simulink model "SS_1115"  (R2014a)
settings: Solver=FixedStepDiscrete  StartTime=0.0  StopTime=5  FixedStep=0.0005  RelTol=1e-3
values from neighbouring files (symbols this model uses):
  APS_High_null = ecucoder_cal(APS_High_null)    [SS.m]
  APS_High_x = ecucoder_cal(APS_High_x)    [SS.m]
  APS_High_y = ecucoder_cal(APS_High_y)    [SS.m]
  APS_Low_null = ecucoder_cal(APS_Low_null)    [SS.m]
  APS_low_x = ecucoder_cal(APS_low_x)    [SS.m]
  APS_low_y = ecucoder_cal(APS_low_y)    [SS.m]
  BrakeSignal_cal = ecucoder_cal(BrakeSignal_cal)    [SS.m]
  CustomReduceFactor_cal = ecucoder_cal(CustomReduceFactor_cal)    [SS.m]
  Differential_cal = ecucoder_cal(Differential_cal)    [SS.m]
  LowSOCWarning_cal = ecucoder_cal(LowSOCWarning_cal)    [SS.m]
  MotorTemperatureHigh_cal = ecucoder_cal(MotorTemperatureHigh_cal)    [SS.m]
  MotorTemperatureLow_cal = ecucoder_cal(MotorTemperatureLow_cal)    [SS.m]
  OilPressure_x = ecucoder_cal(OilPressure_x)    [SS.m]
  OilPressure_y = ecucoder_cal(OilPressure_y)    [SS.m]
  PowerBias_cal = ecucoder_cal(PowerBias_cal)    [SS.m]
  SpeedLimitFactor_x = ecucoder_cal(SpeedLimitFactor_x)    [SS.m]
  SpeedLimitFactor_y = ecucoder_cal(SpeedLimitFactor_y)    [SS.m]
  SteerAngle_x = ecucoder_cal(SteerAngle_x)    [SS.m]
  SteerAngle_y = ecucoder_cal(SteerAngle_y)    [SS.m]
  SteerThresholdHigh_cal = ecucoder_cal(SteerThresholdHigh_cal)    [SS.m]
  SteerThresholdLow_cal = ecucoder_cal(SteerThresholdLow_cal)    [SS.m]
  TorqueLimitNegativ_cal = ecucoder_cal(TorqueLimitNegativ_cal)    [SS.m]
  TorqueLimitPositiv_cal = ecucoder_cal(TorqueLimitPositiv_cal)    [SS.m]
libraries: simulink x101, ec55xxlib x32
(part 3 of 3)

== system SS_1115/VCU_MCU/Enabled Subsystem/Torquearrengement/AMK1 ==
  v : Inport
  Taim : Inport  Port=2
  1-D Lookup Table : Lookup_n-D  NumberOfTableDimensions=1  BreakpointsForDimension1=[0 13000 14000 15000 16000 17000 18000 19000]  Table=[21 21 20 17 16 13 8 0]  ExtrapMethod=Clip  InternalRulePriority=Speed  RndMeth=Simplest  InputSameDT=on
  Constant : Constant  Value=0.0098  SampleTime=-1
  Divide : Product  Inputs=*/  OutDataTypeStr=single
  Divide1 : Product  Inputs=*/  OutDataTypeStr=single
  Saturation : Saturate  UpperLimit=2000  LowerLimit=0
  "ReduceFactor " : Outport
  wires:
  v/1 -> 1-D Lookup Table/1
  1-D Lookup Table/1 -> Divide/1
  Constant/1 -> Divide/2
  Divide/1 -> Saturation/1
  Taim/1 -> Divide1/2
  Divide1/1 -> "ReduceFactor "/1
  Saturation/1 -> Divide1/1

== system SS_1115/VCU_MCU/Enabled Subsystem/Torquearrengement/AMK2 ==
  v : Inport
  Taim : Inport  Port=2
  1-D Lookup Table : Lookup_n-D  NumberOfTableDimensions=1  BreakpointsForDimension1=[0 13000 14000 15000 16000 17000 18000 19000]  Table=[21 21 20 17 16 13 8 0]  ExtrapMethod=Clip  InternalRulePriority=Speed  RndMeth=Simplest  InputSameDT=on
  Constant : Constant  Value=0.0098  SampleTime=-1
  Divide : Product  Inputs=*/  OutDataTypeStr=single
  Divide1 : Product  Inputs=*/  OutDataTypeStr=single
  Saturation : Saturate  UpperLimit=2000  LowerLimit=0
  "ReduceFactor " : Outport
  wires:
  v/1 -> 1-D Lookup Table/1
  1-D Lookup Table/1 -> Divide/1
  Constant/1 -> Divide/2
  Divide/1 -> Saturation/1
  Taim/1 -> Divide1/2
  Divide1/1 -> "ReduceFactor "/1
  Saturation/1 -> Divide1/1

== system SS_1115/VCU_MCU/Enabled Subsystem/Torquearrengement/AMK3 ==
  v : Inport
  Taim : Inport  Port=2
  1-D Lookup Table : Lookup_n-D  NumberOfTableDimensions=1  BreakpointsForDimension1=[0 13000 14000 15000 16000 17000 18000 19000]  Table=[21 21 20 17 16 13 8 0]  ExtrapMethod=Clip  InternalRulePriority=Speed  RndMeth=Simplest  InputSameDT=on
  Constant : Constant  Value=0.0098  SampleTime=-1
  Divide : Product  Inputs=*/  OutDataTypeStr=single
  Divide1 : Product  Inputs=*/  OutDataTypeStr=single
  Saturation : Saturate  UpperLimit=2000  LowerLimit=0
  "ReduceFactor " : Outport
  wires:
  v/1 -> 1-D Lookup Table/1
  1-D Lookup Table/1 -> Divide/1
  Constant/1 -> Divide/2
  Divide/1 -> Saturation/1
  Taim/1 -> Divide1/2
  Divide1/1 -> "ReduceFactor "/1
  Saturation/1 -> Divide1/1

== system SS_1115/VCU_MCU/Enabled Subsystem/Torquearrengement/AMK4 ==
  v : Inport
  Taim : Inport  Port=2
  1-D Lookup Table : Lookup_n-D  NumberOfTableDimensions=1  BreakpointsForDimension1=[0 13000 14000 15000 16000 17000 18000 19000]  Table=[21 21 20 17 16 13 8 0]  ExtrapMethod=Clip  InternalRulePriority=Speed  RndMeth=Simplest  InputSameDT=on
  Constant : Constant  Value=0.0098  SampleTime=-1
  Divide : Product  Inputs=*/  OutDataTypeStr=single
  Divide1 : Product  Inputs=*/  OutDataTypeStr=single
  Saturation : Saturate  UpperLimit=2000  LowerLimit=0
  "ReduceFactor " : Outport
  wires:
  v/1 -> 1-D Lookup Table/1
  1-D Lookup Table/1 -> Divide/1
  Constant/1 -> Divide/2
  Divide/1 -> Saturation/1
  Taim/1 -> Divide1/2
  Divide1/1 -> "ReduceFactor "/1
  Saturation/1 -> Divide1/1

== system SS_1115/VCU_MCU/Enabled Subsystem/Torquearrengement/Differential_ ==
  note: 暂定转角负为左转，正为右转
  note: T1左前 T2右前 T3左后 T4右后
  TIT2 : Inport
  T3T4 : Inport  Port=2
  CAN0333OK : Inport  Port=3
  DifferentialUplimit : Inport  Port=4
  SteerAngleInDegree : Inport  Port=5
  Chart1 : Stateflow chart  TreatAsAtomicUnit=on
  Chart2 : Stateflow chart  TreatAsAtomicUnit=on
  Compare To Constant : simulink/Logic and Bit Operations/Compare To Constant  relop===  const=1  OutDataTypeStr=boolean
  Constant : Constant  Value=SteerThresholdLow_cal  SampleTime=-1
  Constant1 : Constant  Value=SteerThresholdHigh_cal  SampleTime=-1
  Data Type Conversion : DataTypeConversion  OutDataTypeStr=int16
  Data Type Conversion1 : DataTypeConversion  OutDataTypeStr=int16
  Switch : Switch  Criteria=u2 > Threshold
  Unit Delay : UnitDelay  InitialCondition=Differential_cal  SampleTime=-1
  Watchup-Table : Subsystem  TreatAsAtomicUnit=on
  T1 : Outport
  T2 : Outport  Port=2
  T3 : Outport  Port=3
  T4 : Outport  Port=4
  Differential UpLimit : Outport  Port=5
  wires:
  TIT2/1 -> Chart2/1(Sumof2Wheels)
  T3T4/1 -> Chart1/1(Sumof2Wheels)
  CAN0333OK/1 -> Compare To Constant/1
  DifferentialUplimit/1 -> Switch/1
  Unit Delay/1 -> Switch/3
  Compare To Constant/1 -> Switch/2
  Switch/1 -> Unit Delay/1, Watchup-Table/1(DifferentialUpLimit), Differential UpLimit/1  "DifferentialLimit_mea"
  Watchup-Table/1(Differential) -> [DiffFactorRT]  "DiffFactorRT_mea"
  SteerAngleInDegree/1 -> Chart2/2(SteerAngle), Chart1/2(SteerAngle), Watchup-Table/2(SteerAngle)
  Constant/1 -> Data Type Conversion/1
  Data Type Conversion/1 -> Watchup-Table/3(AngleTreshholdLow)  "AngleThresholdLow_mea"
  Constant1/1 -> Data Type Conversion1/1
  Data Type Conversion1/1 -> Watchup-Table/4(AngleTreshholdHigh)  "AngleThresholdHigh_mea"
  [DiffFactorRT] -> Chart2/3(DiffFactorRT)
  Chart2/1(Power2Left) -> T1/1
  Chart2/2(Power2Right) -> T2/1
  Chart1/1(Power2Left) -> T3/1
  Chart1/2(Power2Right) -> T4/1
  [DiffFactorRT] -> Chart1/3(DiffFactorRT)

== system SS_1115/VCU_MCU/Enabled Subsystem/Torquearrengement/Power Cal1 ==
  aim_torque : Inport
  "rotate speed " : Inport  Port=2
  Gain : Gain  Gain=0.0098
  Gain1 : Gain  Gain=1/9549  ParamDataTypeStr=single
  Product : Product  OutDataTypeStr=single
  power : Outport
  wires:
  aim_torque/1 -> Gain/1
  Gain/1 -> Product/1
  "rotate speed "/1 -> Product/2
  Product/1 -> Gain1/1
  Gain1/1 -> power/1

== system SS_1115/VCU_MCU/Enabled Subsystem/Torquearrengement/Power Cal2 ==
  aim_torque : Inport
  "rotate speed " : Inport  Port=2
  Gain : Gain  Gain=0.0098
  Gain1 : Gain  Gain=1/9549  ParamDataTypeStr=single
  Product : Product  OutDataTypeStr=single
  power : Outport
  wires:
  aim_torque/1 -> Gain/1
  Gain/1 -> Product/1
  "rotate speed "/1 -> Product/2
  Product/1 -> Gain1/1
  Gain1/1 -> power/1

== system SS_1115/VCU_MCU/Enabled Subsystem/Torquearrengement/Power Cal3 ==
  aim_torque : Inport
  "rotate speed " : Inport  Port=2
  Gain : Gain  Gain=0.0098
  Gain1 : Gain  Gain=1/9549  ParamDataTypeStr=single
  Product : Product  OutDataTypeStr=single
  power : Outport
  wires:
  aim_torque/1 -> Gain/1
  Gain/1 -> Product/1
  "rotate speed "/1 -> Product/2
  Product/1 -> Gain1/1
  Gain1/1 -> power/1

== system SS_1115/VCU_MCU/Enabled Subsystem/Torquearrengement/Power Cal4 ==
  aim_torque : Inport
  "rotate speed " : Inport  Port=2
  Gain : Gain  Gain=0.0098
  Gain1 : Gain  Gain=1/9549  ParamDataTypeStr=single
  Product : Product  OutDataTypeStr=single
  power : Outport
  wires:
  aim_torque/1 -> Gain/1
  Gain/1 -> Product/1
  "rotate speed "/1 -> Product/2
  Product/1 -> Gain1/1
  Gain1/1 -> power/1

== system SS_1115/VCU_MCU/Enabled Subsystem/Torquearrengement/PowerBias_ ==
  TqSum : Inport
  PowerBias : Inport  Port=2
  CAN0333OK : Inport  Port=3
  Add : Sum  Inputs=+-
  Compare To Constant : simulink/Logic and Bit Operations/Compare To Constant  relop===  const=1  OutDataTypeStr=boolean
  Constant2 : Constant  OutDataTypeStr=single  SampleTime=-1
  Gain : Gain  Gain=80
  Product : Product
  Product1 : Product
  Saturation : Saturate  UpperLimit=1  LowerLimit=0  LinearizeAsGain=off
  Saturation1 : Saturate  UpperLimit=1  LowerLimit=0  LinearizeAsGain=off
  Switch : Switch  Criteria=u2 > Threshold
  Unit Delay : UnitDelay  InitialCondition=PowerBias_cal  SampleTime=-1
  T1T2 : Outport
  T3T4 : Outport  Port=2
  "PowerBias " : Outport  Port=3
  wires:
  TqSum/1 -> Gain/1
  Product/1 -> T1T2/1
  Product1/1 -> T3T4/1
  Add/1 -> Saturation1/1
  [PowerBias] -> Add/2
  Constant2/1 -> Add/1
  CAN0333OK/1 -> Compare To Constant/1
  PowerBias/1 -> Switch/1
  Switch/1 -> [PowerBias], Unit Delay/1
  Unit Delay/1 -> Switch/3
  Compare To Constant/1 -> Switch/2
  [PowerBias] -> "PowerBias "/1
  Gain/1 -> Product1/2, Product/2
  [PowerBias] -> Saturation/1
  Saturation/1 -> Product/1  "FrontPowerBias_mea"
  Saturation1/1 -> Product1/1  "RearPowerBias_mea"

== system SS_1115/HardWare_Input/In1_Message/Function-Call Subsystem/Subsystem1/Subsystem ==
  In1 : Inport
  Bitwise Operator : simulink/Logic and Bit Operations/Bitwise Operator  logicop=AND  UseBitMask=on  BitMask=bin2dec('00000001')  BitMaskRealWorld=Stored Integer
  Bitwise Operator1 : simulink/Logic and Bit Operations/Bitwise Operator  logicop=AND  UseBitMask=on  BitMask=bin2dec('00000010')  BitMaskRealWorld=Stored Integer
  Bitwise Operator2 : simulink/Logic and Bit Operations/Bitwise Operator  logicop=AND  UseBitMask=on  BitMask=bin2dec('00001000')  BitMaskRealWorld=Stored Integer
  Bitwise Operator3 : simulink/Logic and Bit Operations/Bitwise Operator  logicop=AND  UseBitMask=on  BitMask=bin2dec('00100000')  BitMaskRealWorld=Stored Integer
  Shift Arithmetic1 : ArithShift  BitShiftNumber=3  BitShiftDirection=Right
  Shift Arithmetic2 : ArithShift  BitShiftNumber=1  BitShiftDirection=Right
  Shift Arithmetic3 : ArithShift  BitShiftNumber=5  BitShiftDirection=Right
  AMK_bSystemReady : Outport
  AMK_bError : Outport  Port=2
  AMK_bQuitDcOn : Outport  Port=3
  AMK_bQuitInverterOn : Outport  Port=4
  wires:
  Bitwise Operator1/1 -> Shift Arithmetic2/1
  Bitwise Operator/1 -> AMK_bSystemReady/1
  In1/1 -> Bitwise Operator3/1, Bitwise Operator2/1, Bitwise Operator1/1, Bitwise Operator/1
  Shift Arithmetic2/1 -> AMK_bError/1
  Bitwise Operator2/1 -> Shift Arithmetic1/1
  Shift Arithmetic1/1 -> AMK_bQuitDcOn/1
  Bitwise Operator3/1 -> Shift Arithmetic3/1
  Shift Arithmetic3/1 -> AMK_bQuitInverterOn/1

== system SS_1115/HardWare_Input/In2_Message/Function-Call Subsystem/Subsystem1/Subsystem ==
  In1 : Inport
  Bitwise Operator : simulink/Logic and Bit Operations/Bitwise Operator  logicop=AND  UseBitMask=on  BitMask=bin2dec('00000001')  BitMaskRealWorld=Stored Integer
  Bitwise Operator1 : simulink/Logic and Bit Operations/Bitwise Operator  logicop=AND  UseBitMask=on  BitMask=bin2dec('00000010')  BitMaskRealWorld=Stored Integer
  Bitwise Operator2 : simulink/Logic and Bit Operations/Bitwise Operator  logicop=AND  UseBitMask=on  BitMask=bin2dec('00001000')  BitMaskRealWorld=Stored Integer
  Bitwise Operator3 : simulink/Logic and Bit Operations/Bitwise Operator  logicop=AND  UseBitMask=on  BitMask=bin2dec('00100000')  BitMaskRealWorld=Stored Integer
  Shift Arithmetic1 : ArithShift  BitShiftNumber=3  BitShiftDirection=Right
  Shift Arithmetic2 : ArithShift  BitShiftNumber=1  BitShiftDirection=Right
  Shift Arithmetic3 : ArithShift  BitShiftNumber=5  BitShiftDirection=Right
  AMK_bSystemReady : Outport
  AMK_bError : Outport  Port=2
  AMK_bQuitDcOn : Outport  Port=3
  AMK_bQuitInverterOn : Outport  Port=4
  wires:
  Bitwise Operator1/1 -> Shift Arithmetic2/1
  Bitwise Operator/1 -> AMK_bSystemReady/1
  In1/1 -> Bitwise Operator3/1, Bitwise Operator2/1, Bitwise Operator1/1, Bitwise Operator/1
  Shift Arithmetic2/1 -> AMK_bError/1
  Bitwise Operator2/1 -> Shift Arithmetic1/1
  Shift Arithmetic1/1 -> AMK_bQuitDcOn/1
  Bitwise Operator3/1 -> Shift Arithmetic3/1
  Shift Arithmetic3/1 -> AMK_bQuitInverterOn/1

== system SS_1115/HardWare_Input/In3_Message/Function-Call Subsystem/Subsystem1/Subsystem ==
  In1 : Inport
  Bitwise Operator : simulink/Logic and Bit Operations/Bitwise Operator  logicop=AND  UseBitMask=on  BitMask=bin2dec('00000001')  BitMaskRealWorld=Stored Integer
  Bitwise Operator1 : simulink/Logic and Bit Operations/Bitwise Operator  logicop=AND  UseBitMask=on  BitMask=bin2dec('00000010')  BitMaskRealWorld=Stored Integer
  Bitwise Operator2 : simulink/Logic and Bit Operations/Bitwise Operator  logicop=AND  UseBitMask=on  BitMask=bin2dec('00001000')  BitMaskRealWorld=Stored Integer
  Bitwise Operator3 : simulink/Logic and Bit Operations/Bitwise Operator  logicop=AND  UseBitMask=on  BitMask=bin2dec('00100000')  BitMaskRealWorld=Stored Integer
  Shift Arithmetic1 : ArithShift  BitShiftNumber=3  BitShiftDirection=Right
  Shift Arithmetic2 : ArithShift  BitShiftNumber=1  BitShiftDirection=Right
  Shift Arithmetic3 : ArithShift  BitShiftNumber=5  BitShiftDirection=Right
  AMK_bSystemReady : Outport
  AMK_bError : Outport  Port=2
  AMK_bQuitDcOn : Outport  Port=3
  AMK_bQuitInverterOn : Outport  Port=4
  wires:
  Bitwise Operator1/1 -> Shift Arithmetic2/1
  Bitwise Operator/1 -> AMK_bSystemReady/1
  In1/1 -> Bitwise Operator3/1, Bitwise Operator2/1, Bitwise Operator1/1, Bitwise Operator/1
  Shift Arithmetic2/1 -> AMK_bError/1
  Bitwise Operator2/1 -> Shift Arithmetic1/1
  Shift Arithmetic1/1 -> AMK_bQuitDcOn/1
  Bitwise Operator3/1 -> Shift Arithmetic3/1
  Shift Arithmetic3/1 -> AMK_bQuitInverterOn/1

== system SS_1115/HardWare_Input/In4_Message/Function-Call Subsystem/Subsystem1/Subsystem ==
  In1 : Inport
  Bitwise Operator : simulink/Logic and Bit Operations/Bitwise Operator  logicop=AND  UseBitMask=on  BitMask=bin2dec('00000001')  BitMaskRealWorld=Stored Integer
  Bitwise Operator1 : simulink/Logic and Bit Operations/Bitwise Operator  logicop=AND  UseBitMask=on  BitMask=bin2dec('00000010')  BitMaskRealWorld=Stored Integer
  Bitwise Operator2 : simulink/Logic and Bit Operations/Bitwise Operator  logicop=AND  UseBitMask=on  BitMask=bin2dec('00001000')  BitMaskRealWorld=Stored Integer
  Bitwise Operator3 : simulink/Logic and Bit Operations/Bitwise Operator  logicop=AND  UseBitMask=on  BitMask=bin2dec('00100000')  BitMaskRealWorld=Stored Integer
  Shift Arithmetic1 : ArithShift  BitShiftNumber=3  BitShiftDirection=Right
  Shift Arithmetic2 : ArithShift  BitShiftNumber=1  BitShiftDirection=Right
  Shift Arithmetic3 : ArithShift  BitShiftNumber=5  BitShiftDirection=Right
  AMK_bSystemReady : Outport
  AMK_bError : Outport  Port=2
  AMK_bQuitDcOn : Outport  Port=3
  AMK_bQuitInverterOn : Outport  Port=4
  wires:
  Bitwise Operator1/1 -> Shift Arithmetic2/1
  Bitwise Operator/1 -> AMK_bSystemReady/1
  In1/1 -> Bitwise Operator3/1, Bitwise Operator2/1, Bitwise Operator1/1, Bitwise Operator/1
  Shift Arithmetic2/1 -> AMK_bError/1
  Bitwise Operator2/1 -> Shift Arithmetic1/1
  Shift Arithmetic1/1 -> AMK_bQuitDcOn/1
  Bitwise Operator3/1 -> Shift Arithmetic3/1
  Shift Arithmetic3/1 -> AMK_bQuitInverterOn/1

== system SS_1115/VCU_MCU/Enabled Subsystem/Torquearrengement/Differential_/Watchup-Table ==
  DifferentialUpLimit : Inport
  SteerAngle : Inport  Port=2
  AngleTreshholdLow : Inport  Port=3
  AngleTreshholdHigh : Inport  Port=4
  Abs : Abs
  Chart : Stateflow chart  TreatAsAtomicUnit=on
  Saturation : Saturate  UpperLimit=1  LowerLimit=0  LinearizeAsGain=off
  Differential : Outport
  wires:
  DifferentialUpLimit/1 -> Chart/1(DiffLimit)
  SteerAngle/1 -> Abs/1
  AngleTreshholdHigh/1 -> Chart/4(ThresholdHigh)
  AngleTreshholdLow/1 -> Chart/3(ThresholdLow)
  Chart/1(DiffFactor) -> Saturation/1
  Abs/1 -> Chart/2(SteerAngle)
  Saturation/1 -> Differential/1

== stateflow chart SS_1115/VCU_MCU/Enabled Subsystem/Chart1 ==
  state Normal
    entry:
    Logicvalue = single(1);
  state TimeCounting
    entry:
    Logicvalue = single(1);
  state Warning
    entry:
    Logicvalue = single(0);
  (default) -> Normal
  Warning -> Normal : [APPS_PCT<=5]
  Normal -> TimeCounting : [BrakeSignal==1&APPS_PCT>=15]
  TimeCounting -> Normal [order 1] : [BrakeSignal==0||APPS_PCT<15]
  TimeCounting -> Warning [order 2] : after(40,tick)
  data: BrakeSignal input; APPS_PCT input; Logicvalue output

== stateflow chart SS_1115/VCU_MCU/Enabled Subsystem/DRS Strategy ==
  state DRSOFF
    entry:
    DRSState=uint8(0);
  state DRSON
    entry:
    DRSState=uint8(1);
  (default) -> DRSOFF
  DRSOFF -> DRSON : [DRSCMD==1&&BrakeSignal==0]
  DRSON -> DRSOFF : [DRSCMD==0||BrakeSignal==1]
  data: BrakeSignal input; DRSCMD input; DRSState output

== stateflow chart SS_1115/VCU_MCU/Enabled Subsystem/Torquearrengement/Chart ==
  (default) -> (junction 6)
  (junction 6) -> (junction 5) [order 1] : [powersum<=53.3]
  (junction 6) -> (junction 7) [order 2] : {factor=single(53.3/powersum);}
  (junction 5) -> (junction 4) : {factor=single(1);}
  (junction 4) -> (junction 7)
  (junction 7) -> (junction 3)
  data: powersum input single; factor output single

== stateflow chart SS_1115/VCU_MCU/Enabled Subsystem/Torquearrengement/Differential_/Watchup-Table/Chart ==
  state DiffON
    entry:
    DiffFactor = single(DiffLimit*((SteerAngle-ThresholdLow)/(ThresholdHigh-ThresholdLow)));
  state FullDiff
    entry:
    DiffFactor = single(1);
  state Default
    entry:
    DiffFactor = single(0);
  (default) -> Default
  Default -> DiffON [order 2] : [SteerAngle<=ThresholdLow]
  DiffON -> FullDiff : [SteerAngle>=ThresholdHigh]
  FullDiff -> DiffON : [SteerAngle<ThresholdHigh]
  Default -> DiffON [order 1] : [SteerAngle>ThresholdLow && SteerAngle<ThresholdHigh]
  data: DiffLimit input; SteerAngle input; ThresholdLow input; ThresholdHigh input; DiffFactor output

== stateflow chart SS_1115/VCU_MCU/Enabled Subsystem/Torquearrengement/Differential_/Chart2 ==
  state SteerLeft
    entry:
    Power2Left = single(0.5*(1-DiffFactorRT)*Sumof2Wheels);
    Power2Right = single(0.5*(1+DiffFactorRT)*Sumof2Wheels);
  state SteerRight
    entry:
    Power2Left = single(0.5*(1+DiffFactorRT)*Sumof2Wheels);
    Power2Right = single(0.5*(1-DiffFactorRT)*Sumof2Wheels);
  (default) -> SteerLeft
  SteerLeft -> SteerRight : [SteerAngle>=0]
  SteerRight -> SteerLeft : [SteerAngle<0]
  data: Sumof2Wheels input; SteerAngle input; DiffFactorRT input; Power2Left output; Power2Right output

== stateflow chart SS_1115/VCU_MCU/Enabled Subsystem/BuzzingLogic ==
  state Standby
    entry:
    AMK_InverterOn=uint8(1);
    AMK_DcOn= uint8(1);
    AMK_Enable= uint8(0);
    AMK_ErrorReset= uint8(0);
    AMK_TorqueLimitPositiv= int16(0);
    AMK_TorqueLimitNegativ= int16(0);
    Buzzing= uint8(0);
  state Running
    entry:
    AMK_InverterOn=uint8(1);
    AMK_DcOn= uint8(1);
    AMK_Enable= uint8(1);
    AMK_ErrorReset= uint8(0);
    AMK_TorqueLimitPositiv=int16(TorqueLimitPositiv_cal);
    AMK_TorqueLimitNegativ=int16(TorqueLimitNegativ_cal);
    Buzzing= uint8(0);
  state BrakeStandby
    entry:
    AMK_InverterOn=uint8(1);
    AMK_DcOn=uint8(1);
    AMK_Enable=uint8(0);
    AMK_ErrorReset=uint8(0);
    AMK_TorqueLimitPositiv=int16(0);
    AMK_TorqueLimitNegativ=int16(0);
    Buzzing=uint8(0);
  state MotorSpeedReq
    entry:
    AMK_InverterOn=uint8(1);
    AMK_DcOn=uint8(1);
    AMK_Enable=uint8(0);
    AMK_ErrorReset=uint8(0);
    AMK_TorqueLimitPositiv=int16(0);
    AMK_TorqueLimitNegativ=int16(0);
    Buzzing= uint8(0);
  state Buzzing
    entry:
    AMK_InverterOn=uint8(1);
    AMK_DcOn= uint8(1);
    AMK_Enable= uint8(1);
    AMK_ErrorReset= uint8(0);
    AMK_TorqueLimitPositiv= int16(0);
    AMK_TorqueLimitNegativ= int16(0);
    Buzzing= uint8(1);
  (default) -> Standby
  Running -> Standby : [StartSignal==0]
  Standby -> BrakeStandby : [BrakeSignal==1&StartSignal==0]
  BrakeStandby -> Standby [order 2] : [StartSignal==1&BrakeSignal==0]
  Buzzing -> Running : after(200,tick)
  BrakeStandby -> MotorSpeedReq [order 1] : [BrakeSignal==1&StartSignal==1]
  MotorSpeedReq -> Buzzing : after(100,tick)
  data: AMK_InverterOn output uint8; AMK_DcOn output uint8; AMK_Enable output uint8; AMK_ErrorReset output uint8; AMK_TorqueLimitPositiv output int16; AMK_TorqueLimitNegativ output int16; StartSignal input boolean; Buzzing output uint8; BrakeSignal input boolean; TorqueLimitPositiv_cal input; TorqueLimitNegativ_cal input

== stateflow chart SS_1115/VCU_MCU/Enabled Subsystem/Torquearrengement/Differential_/Chart1 ==
  state SteerLeft
    entry:
    Power2Left = single(0.5*(1-DiffFactorRT)*Sumof2Wheels);
    Power2Right = single(0.5*(1+DiffFactorRT)*Sumof2Wheels);
  state SteerRight
    entry:
    Power2Left = single(0.5*(1+DiffFactorRT)*Sumof2Wheels);
    Power2Right = single(0.5*(1-DiffFactorRT)*Sumof2Wheels);
  (default) -> SteerLeft
  SteerLeft -> SteerRight : [SteerAngle>=0]
  SteerRight -> SteerLeft : [SteerAngle<0]
  data: Sumof2Wheels input; SteerAngle input; DiffFactorRT input; Power2Left output; Power2Right output
